simulink model "upDownCounter"  (R2023b)
settings: Solver=FixedStepAuto  StartTime=0.0  StopTime=100  FixedStep=1  RelTol=1e-3
undefined symbols (not defined in the file or in its folder): DiscIntNeverNeededParam
settings Model: Creator=z004f2se  LastModifiedBy=z004f2se

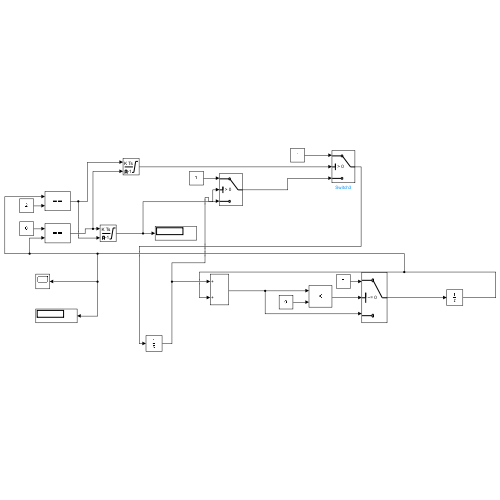
[thumbnail: Simulink's stored preview of the top-level diagram]
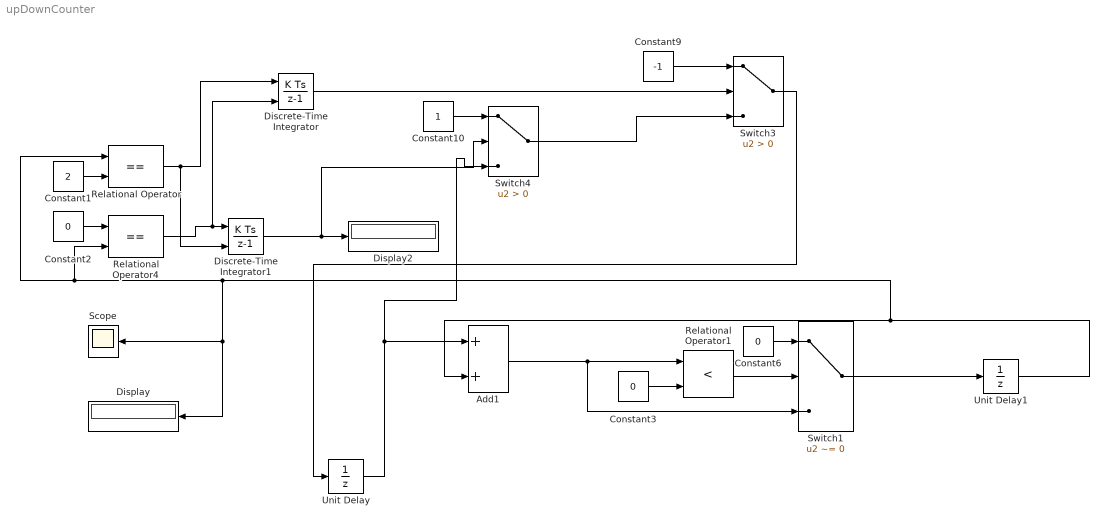
== system upDownCounter ==
  Add1 : Sum
  Constant1 : Constant  Value=2  SampleTime=-1
  Constant10 : Constant
  Constant2 : Constant  Value=0  SampleTime=-1
  Constant3 : Constant  Value=0  SampleTime=-1
  Constant6 : Constant  Value=0  SampleTime=-1
  Constant9 : Constant  Value=-1
  Discrete-Time Integrator : DiscreteIntegrator  ExternalReset=level  SampleTime=-1  OutDataTypeStr=double  LimitOutput=on  UpperSaturationLimit=1  ICPrevOutput=DiscIntNeverNeededParam  ICPrevScaledInput=DiscIntNeverNeededParam
  Discrete-Time Integrator1 : DiscreteIntegrator  ExternalReset=level  SampleTime=-1  OutDataTypeStr=double  LimitOutput=on  UpperSaturationLimit=1  ICPrevOutput=DiscIntNeverNeededParam  ICPrevScaledInput=DiscIntNeverNeededParam
  Display : Display
  Display2 : Display
  Relational Operator : RelationalOperator  Operator===  OutDataTypeStr=boolean  RndMeth=Simplest  InputSameDT=off
  Relational Operator1 : RelationalOperator  Operator=<  OutDataTypeStr=boolean  RndMeth=Simplest  InputSameDT=off
  Relational Operator4 : RelationalOperator  Operator===  OutDataTypeStr=boolean  RndMeth=Simplest  InputSameDT=off
  Scope : Scope
  Switch1 : Switch  Criteria=u2 ~= 0  SaturateOnIntegerOverflow=off  InputSameDT=off
  Switch3 : Switch  Criteria=u2 > Threshold  SaturateOnIntegerOverflow=off  InputSameDT=off
  Switch4 : Switch  Criteria=u2 > Threshold  SaturateOnIntegerOverflow=off  InputSameDT=off
  Unit Delay : UnitDelay  SampleTime=-1  HasFrameUpgradeWarning=on
  Unit Delay1 : UnitDelay  SampleTime=-1  HasFrameUpgradeWarning=on
  wires:
  Constant1/1 -> Relational Operator/2
  Unit Delay/1 -> Switch4/3, Add1/1
  Unit Delay1/1 -> Add1/2, Display/1, Scope/1, Relational Operator4/2, Relational Operator/1
  Relational Operator/1 -> Discrete-Time Integrator1/2, Discrete-Time Integrator/1
  Discrete-Time Integrator1/1 -> Switch4/2, Display2/1
  Discrete-Time Integrator/1 -> Switch3/2
  Constant2/1 -> Relational Operator4/1
  Relational Operator4/1 -> Discrete-Time Integrator/2, Discrete-Time Integrator1/1
  Constant9/1 -> Switch3/1
  Constant10/1 -> Switch4/1
  Switch3/1 -> Unit Delay/1
  Switch4/1 -> Switch3/3
  Constant3/1 -> Relational Operator1/2
  Add1/1 -> Switch1/3, Relational Operator1/1
  Relational Operator1/1 -> Switch1/2
  Switch1/1 -> Unit Delay1/1
  Constant6/1 -> Switch1/1
